simulink model "RomiRLSim_v1"  (R2020b)
settings: Solver=VariableStepAuto  StartTime=0.0  StopTime=1000  RelTol=1e-3
model workspace (MAT data in the model file):
  max_speed = Simulink.Parameter
  max_speed.Value = 2
  max_speed.DataType = 'auto'
  max_speed.Dimensions = [1 1]
values from neighbouring files (symbols this model uses):
  max_speed = 2    [parameters.m]
  Ts = 0.025    [parameters.m]
  waypoint = [1,1]    [parameters.m]    (also in romi_reset_fn.m = round([r * cos(deg), r * sin(deg)], 2))
libraries: simulink x5, mobileRoboticsLib x2, rllib x1
settings Model: Creator=91819  LastModifiedBy=91819

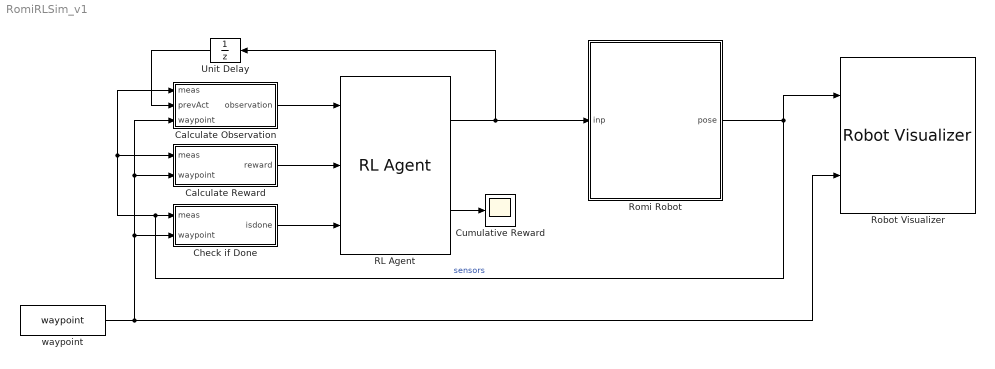
== system RomiRLSim_v1 ==
  Calculate Observation : Subsystem
  Calculate Reward : Subsystem
  Check if Done : Subsystem
  Cumulative Reward : Scope
  RL Agent : rllib/RL Agent  Agent=agent  ProvideReward=on  ProvideIsDone=on  ProvideCumRwd=on  TreatAsDirectFeedthrough=on  CollectLoggedSignals=on  CollectModelStates=on
      settings: SourceProductName=Reinforcement Learning
  Robot Visualizer : mobileRoboticsLib/Environments/Robot Visualizer  Priority=99  robotRadius=0  showTrajectory=on  hasWaypoints=on  hasLidar=off  sensorOffset=[ 0 0 ]  scanAngles=0  hasObjDetector=off  objDetectorOffset=[ 0, 0 ]  objDetectorAngle=0  objDetectorFOV=0  objDetectorMaxRange=0  objectColors=0  objectMarkers=s
      settings: SourceProductName=Ground Vehicles Library
  Romi Robot : Subsystem
  Unit Delay : UnitDelay  SampleTime=-1  HasFrameUpgradeWarning=on
  waypoint : Constant  Value=waypoint  VectorParams1D=off
  wires:
  Calculate Reward/1(reward) -> RL Agent/2
  Calculate Observation/1(observation) -> RL Agent/1
  RL Agent/1 -> Romi Robot/1(inp), Unit Delay/1
  RL Agent/2 -> Cumulative Reward/1
  Unit Delay/1 -> Calculate Observation/2(prevAct)
  Check if Done/1(isdone) -> RL Agent/3
  Romi Robot/1(pose) -> Calculate Reward/1(meas), Calculate Observation/1(meas), Check if Done/1(meas), Robot Visualizer/1  "sensors"
  waypoint/1 -> Robot Visualizer/2, Check if Done/2(waypoint), Calculate Reward/2(waypoint), Calculate Observation/3(waypoint)

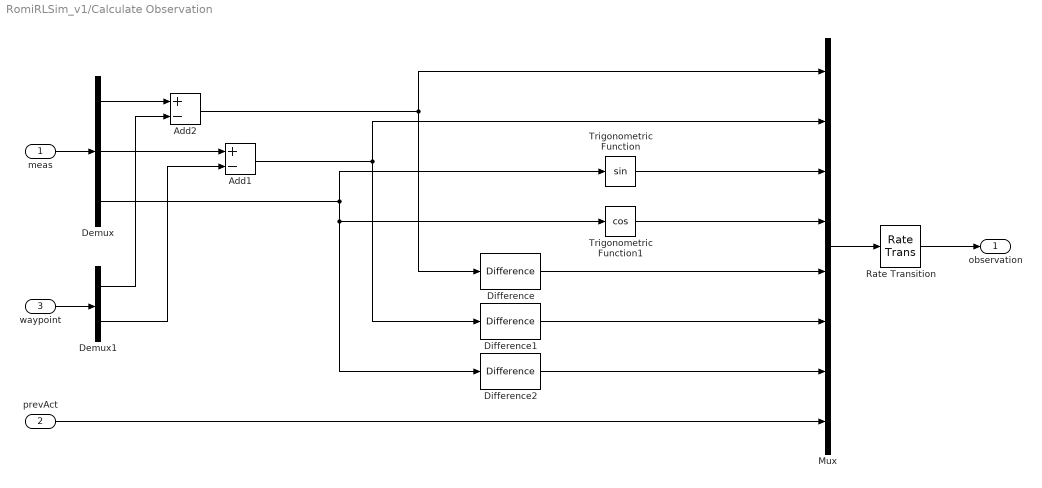
== system RomiRLSim_v1/Calculate Observation ==
  meas : Inport
  prevAct : Inport  Port=2
  waypoint : Inport  Port=3
  Add1 : Sum  Inputs=+-
  Add2 : Sum  Inputs=+-
  Demux : Demux  Outputs=3
  Demux1 : Demux  Outputs=2
  Difference : simulink/Discrete/Difference  ICPrevInput=0.0  OutMin=[]  OutMax=[]  OutDataType=fixdt(1, 16)  OutScaling=2^-10  DoSatur=off
  Difference1 : simulink/Discrete/Difference  ICPrevInput=0.0  OutMin=[]  OutMax=[]  OutDataType=fixdt(1, 16)  OutScaling=2^-10  DoSatur=off
  Difference2 : simulink/Discrete/Difference  ICPrevInput=0.0  OutMin=[]  OutMax=[]  OutDataType=fixdt(1, 16)  OutScaling=2^-10  DoSatur=off
  Mux : Mux  Inputs=8
  Rate Transition : RateTransition
  Trigonometric Function : Trigonometry
  Trigonometric Function1 : Trigonometry  Operator=cos
  observation : Outport  VectorParamsAs1DForOutWhenUnconnected=off
  wires:
  meas/1 -> Demux/1
  Mux/1 -> Rate Transition/1
  Rate Transition/1 -> observation/1
  prevAct/1 -> Mux/8
  Add2/1 -> Difference/1, Mux/1
  Add1/1 -> Mux/2, Difference1/1
  Demux/3 -> Trigonometric Function1/1, Difference2/1, Trigonometric Function/1
  Difference/1 -> Mux/5
  Difference1/1 -> Mux/6
  Difference2/1 -> Mux/7
  waypoint/1 -> Demux1/1
  Demux/1 -> Add2/1
  Demux1/1 -> Add2/2
  Demux/2 -> Add1/1
  Demux1/2 -> Add1/2
  Trigonometric Function/1 -> Mux/3
  Trigonometric Function1/1 -> Mux/4

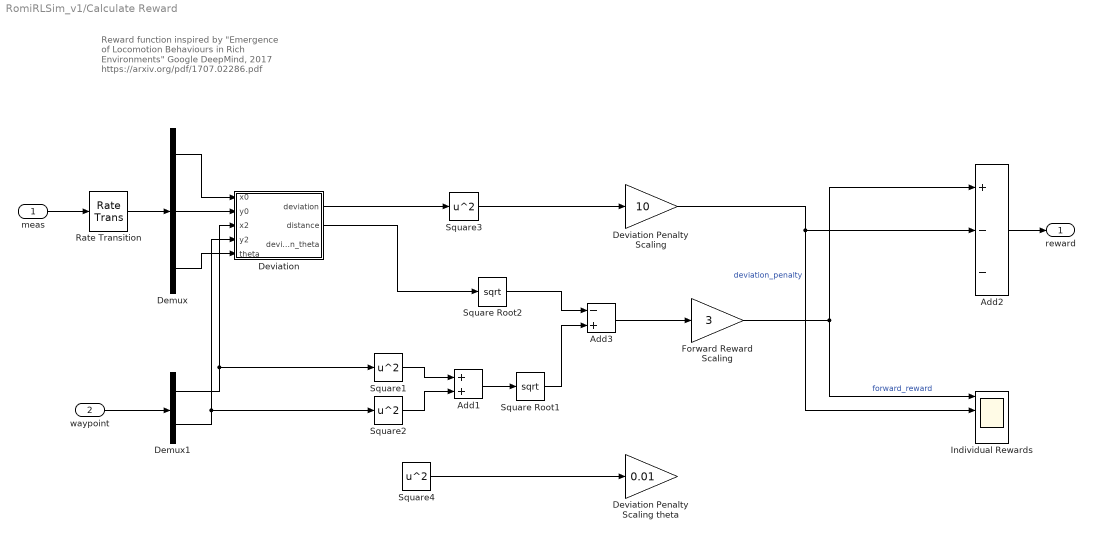
== system RomiRLSim_v1/Calculate Reward ==
  note: Reward function inspired by
      | "Emergence of Locomotion Behaviours in Rich Environments"
      | Google DeepMind, 2017
      | https://arxiv.org/pdf/1707.02286.pdf
  meas : Inport
  waypoint : Inport  Port=2
  Add1 : Sum
  Add2 : Sum  Inputs=+--
  Add3 : Sum  Inputs=-+
  Demux : Demux  Outputs=3
  Demux1 : Demux  Outputs=2
  Deviation : Subsystem
  Deviation Penalty Scaling : Gain  Gain=10
  Deviation Penalty Scaling theta : Gain  Gain=0.01
  Forward Reward Scaling : Gain  Gain=3
  Individual Rewards : Scope  NumInputPorts=4
  Rate Transition : RateTransition  OutPortSampleTime=Ts
  Square Root1 : Sqrt  SaturateOnIntegerOverflow=on
  Square Root2 : Sqrt  SaturateOnIntegerOverflow=on
  Square1 : Math  Operator=square  SaturateOnIntegerOverflow=on
  Square2 : Math  Operator=square  SaturateOnIntegerOverflow=on
  Square3 : Math  Operator=square  SignedPower=on  SaturateOnIntegerOverflow=on
  Square4 : Math  Operator=square  SignedPower=on  SaturateOnIntegerOverflow=on
  reward : Outport  VectorParamsAs1DForOutWhenUnconnected=off
  wires:
  meas/1 -> Rate Transition/1
  Rate Transition/1 -> Demux/1
  Add2/1 -> reward/1
  Deviation Penalty Scaling/1 -> Individual Rewards/2, Add2/2  "deviation_penalty"
  Forward Reward Scaling/1 -> Add2/1, Individual Rewards/1  "forward_reward"
  Demux/2 -> Deviation/2(y0)
  waypoint/1 -> Demux1/1
  Deviation/1(deviation) -> Square3/1
  Demux/1 -> Deviation/1(x0)
  Deviation/2(distance) -> Square Root2/1
  Square Root2/1 -> Add3/1
  Add1/1 -> Square Root1/1
  Demux1/1 -> Square1/1, Deviation/3(x2)
  Square Root1/1 -> Add3/2
  Demux1/2 -> Square2/1, Deviation/4(y2)
  Square1/1 -> Add1/1
  Square2/1 -> Add1/2
  Add3/1 -> Forward Reward Scaling/1
  Demux/3 -> Deviation/5(theta)
  Square3/1 -> Deviation Penalty Scaling/1
  Square4/1 -> Deviation Penalty Scaling theta/1

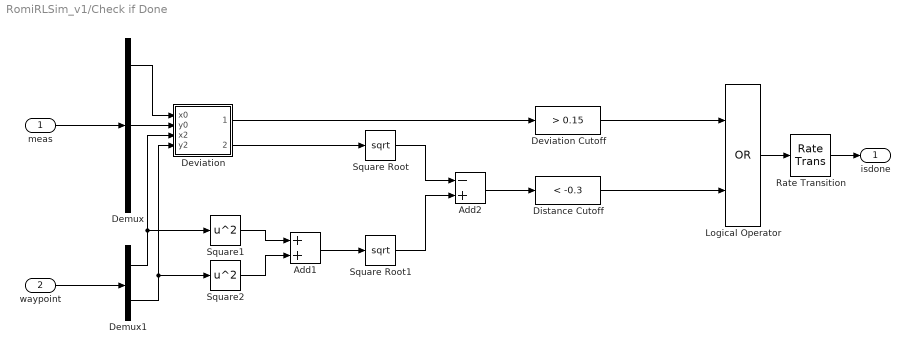
== system RomiRLSim_v1/Check if Done ==
  meas : Inport
  waypoint : Inport  Port=2
  Add1 : Sum
  Add2 : Sum  Inputs=-+
  Demux : Demux  Outputs=3
  Demux1 : Demux  Outputs=2
  Deviation : Subsystem
  Deviation Cutoff : simulink/Logic and Bit Operations/Compare To Constant  relop=>  const=0.15  OutDataTypeStr=boolean
  Distance Cutoff : simulink/Logic and Bit Operations/Compare To Constant  relop=<  const=-0.3  OutDataTypeStr=boolean
  Logical Operator : Logic  Operator=OR  AllPortsSameDT=off  OutDataTypeStr=boolean
  Rate Transition : RateTransition
  Square Root : Sqrt  SaturateOnIntegerOverflow=on
  Square Root1 : Sqrt  SaturateOnIntegerOverflow=on
  Square1 : Math  Operator=square  SaturateOnIntegerOverflow=on
  Square2 : Math  Operator=square  SaturateOnIntegerOverflow=on
  isdone : Outport  VectorParamsAs1DForOutWhenUnconnected=off
  wires:
  Logical Operator/1 -> Rate Transition/1
  Rate Transition/1 -> isdone/1
  Deviation Cutoff/1 -> Logical Operator/1
  Demux/2 -> Deviation/2(y0)
  meas/1 -> Demux/1
  Demux1/2 -> Square2/1, Deviation/4(y2)
  Demux1/1 -> Square1/1, Deviation/3(x2)
  Demux/1 -> Deviation/1(x0)
  waypoint/1 -> Demux1/1
  Deviation/1(deviation) -> Deviation Cutoff/1
  Deviation/2(distance) -> Square Root/1
  Add1/1 -> Square Root1/1
  Square1/1 -> Add1/1
  Square2/1 -> Add1/2
  Square Root/1 -> Add2/1
  Square Root1/1 -> Add2/2
  Add2/1 -> Distance Cutoff/1
  Distance Cutoff/1 -> Logical Operator/2

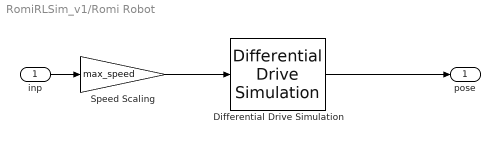
== system RomiRLSim_v1/Romi Robot ==
  inp : Inport
  Differential Drive Simulation : mobileRoboticsLib/Kinematic Models/Differential Drive/Differential Drive Simulation  wheelRadius=0.035  wheelBase=0.145  initX=x0  initY=y0  initAngle=theta0  Ts=Ts
      settings: SourceProductName=Mobile Robotics Simulation Toolbox
  Speed Scaling : Gain  Gain=max_speed
  pose : Outport  VectorParamsAs1DForOutWhenUnconnected=off
  wires:
  inp/1 -> Speed Scaling/1
  Speed Scaling/1 -> Differential Drive Simulation/1
  Differential Drive Simulation/1 -> pose/1

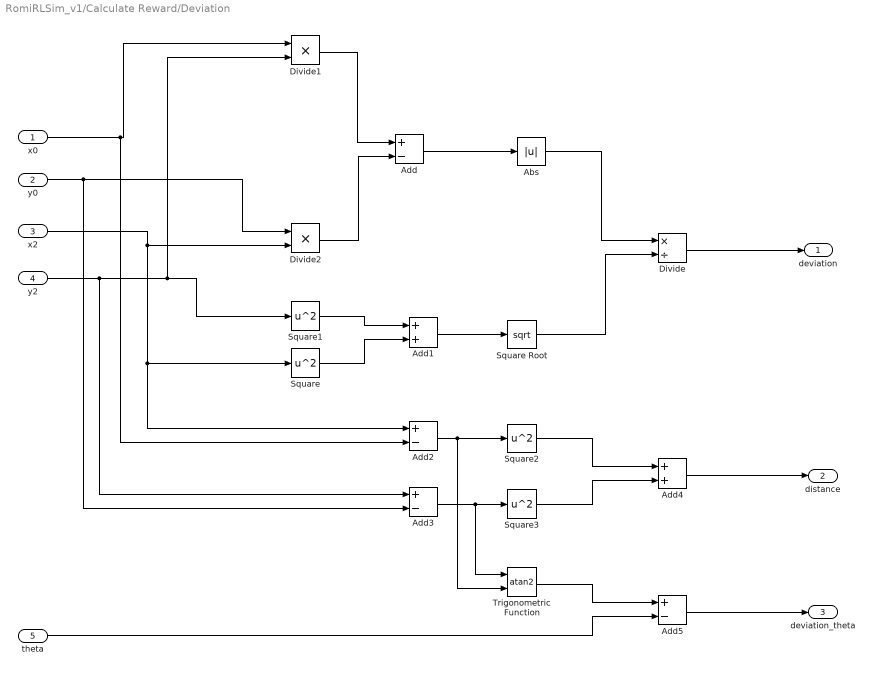
== system RomiRLSim_v1/Calculate Reward/Deviation ==
  x0 : Inport
  y0 : Inport  Port=2
  x2 : Inport  Port=3
  y2 : Inport  Port=4
  theta : Inport  Port=5
  Abs : Abs
  Add{,2..3,5} (4 alike) : Sum  Inputs=+-
  Add1 : Sum
  Add4 : Sum
  Divide : Product  Inputs=*/
  Divide1 : Product  Inputs=**
  Divide2 : Product  Inputs=**
  Square{,1..3} (4 alike) : Math  Operator=square  SaturateOnIntegerOverflow=on
  Square Root : Sqrt  SaturateOnIntegerOverflow=on
  Trigonometric Function : Trigonometry  Operator=atan2
  deviation : Outport
  distance : Outport  Port=2
  deviation_theta : Outport  Port=3
  wires:
  x0/1 -> Divide1/1, Add2/2
  y0/1 -> Divide2/1, Add3/2
  y2/1 -> Divide1/2, Square1/1, Add3/1
  Divide1/1 -> Add/1
  Divide2/1 -> Add/2
  Add/1 -> Abs/1
  x2/1 -> Divide2/2, Add2/1, Square/1
  Square1/1 -> Add1/1
  Square/1 -> Add1/2
  Add1/1 -> Square Root/1
  Abs/1 -> Divide/1
  Square Root/1 -> Divide/2
  Divide/1 -> deviation/1
  Add2/1 -> Trigonometric Function/2, Square2/1
  Add4/1 -> distance/1
  Square2/1 -> Add4/1
  Square3/1 -> Add4/2
  theta/1 -> Add5/2
  Trigonometric Function/1 -> Add5/1
  Add5/1 -> deviation_theta/1
  Add3/1 -> Trigonometric Function/1, Square3/1

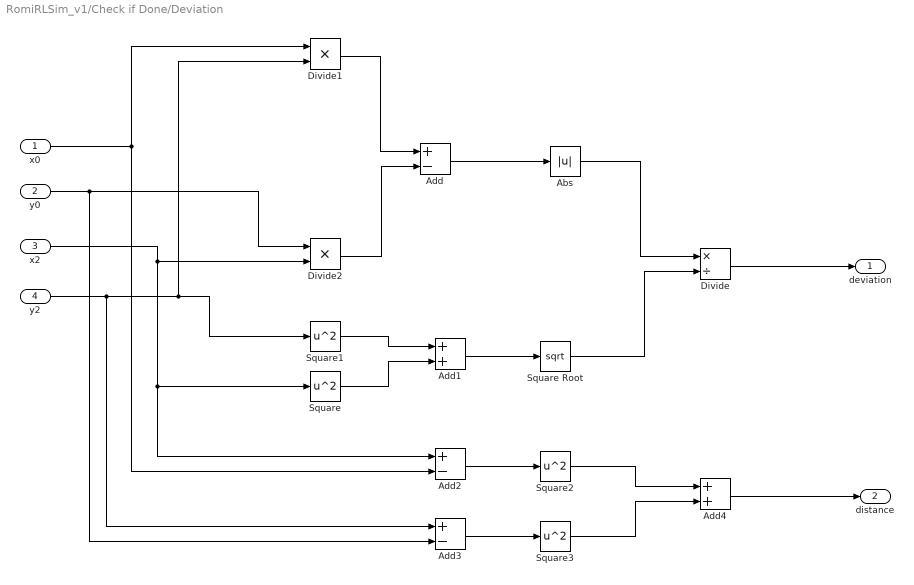
== system RomiRLSim_v1/Check if Done/Deviation ==
  x0 : Inport
  y0 : Inport  Port=2
  x2 : Inport  Port=3
  y2 : Inport  Port=4
  Abs : Abs
  Add : Sum  Inputs=+-
  Add1 : Sum
  Add2 : Sum  Inputs=+-
  Add3 : Sum  Inputs=+-
  Add4 : Sum
  Divide : Product  Inputs=*/
  Divide1 : Product  Inputs=**
  Divide2 : Product  Inputs=**
  Square{,1..3} (4 alike) : Math  Operator=square  SaturateOnIntegerOverflow=on
  Square Root : Sqrt  SaturateOnIntegerOverflow=on
  deviation : Outport
  distance : Outport  Port=2
  wires:
  x0/1 -> Divide1/1, Add2/2
  y0/1 -> Divide2/1, Add3/2
  y2/1 -> Divide1/2, Square1/1, Add3/1
  Divide1/1 -> Add/1
  Divide2/1 -> Add/2
  Add/1 -> Abs/1
  x2/1 -> Divide2/2, Add2/1, Square/1
  Square1/1 -> Add1/1
  Square/1 -> Add1/2
  Add1/1 -> Square Root/1
  Abs/1 -> Divide/1
  Square Root/1 -> Divide/2
  Divide/1 -> deviation/1
  Add2/1 -> Square2/1
  Add3/1 -> Square3/1
  Add4/1 -> distance/1
  Square2/1 -> Add4/1
  Square3/1 -> Add4/2
